simulink model "Bitwise_Testing"  (R2019a)
settings: Solver=FixedStepDiscrete  StartTime=0.0  StopTime=10.0  RelTol=1e-3
libraries: simulink x3
settings Model: Creator=Raouf  LastModifiedBy=Raouf
settings OptimizationCC: DefaultParameterBehavior=Inlined  EnhancedBackFolding=on  PassReuseOutputArgsAs=Individual arguments  OptimizeBlockOrder=speed  DifferentSizesBufferReuse=on  OptimizationCustomize=off
settings DebuggingCC: ParameterTunabilityLossMsg=error
settings SFSimCC: MATLABDynamicMemAlloc=off
settings RTWCC: SystemTargetFile=ert.tlc  GenCodeOnly=on  TemplateMakefile=ert_default_tmf  GenerateReport=on  IncludeHyperlinkInReport=on  LaunchReport=on  GenerateTraceInfo=on  GenerateTraceReport=on  GenerateTraceReportSl=on  GenerateTraceReportSf=on  GenerateTraceReportEml=on
settings CodeAppCC: ForceParamTrailComments=on  IgnoreCustomStorageClasses=off  OperatorAnnotations=on  SimulinkDataObjDesc=on  SFDataObjDesc=on  InsertBlockDesc=on
settings ERTTargetCC: TargetLangStandard=C99 (ISO)  GenerateSampleERTMain=on  InlinedParameterPlacement=NonHierarchical  ERTCustomFileTemplate=example_file_process.tlc

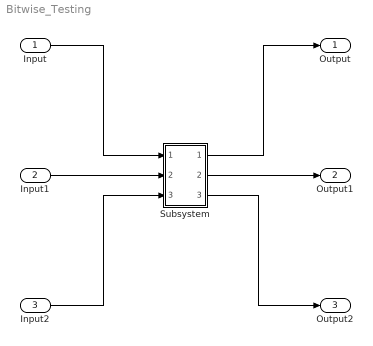
== system Bitwise_Testing ==
  Input : Inport  OutDataTypeStr=uint8
  Input1 : Inport  Port=2  OutDataTypeStr=uint8
  Input2 : Inport  Port=3  OutDataTypeStr=uint8
  Subsystem : Subsystem
  Output : Outport
  Output1 : Outport  Port=2
  Output2 : Outport  Port=3
  wires:
  Input/1 -> Subsystem/1(In1)
  Input1/1 -> Subsystem/2(In2)
  Input2/1 -> Subsystem/3(In3)
  Subsystem/1(Out1) -> Output/1
  Subsystem/2(Out2) -> Output1/1
  Subsystem/3(Out3) -> Output2/1

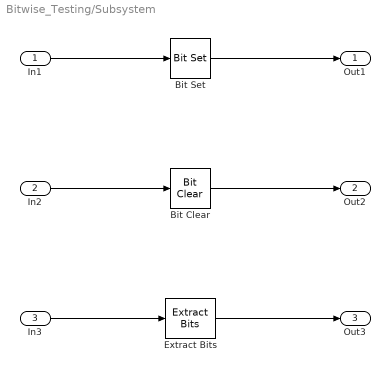
== system Bitwise_Testing/Subsystem ==
  In1 : Inport
  In2 : Inport  Port=2
  In3 : Inport  Port=3
  Bit Clear : simulink/Logic and Bit Operations/Bit Clear  iBit=0
      settings: SourceProductName=Simulink  SourceProductBaseCode=SL
  Bit Set : simulink/Logic and Bit Operations/Bit Set  iBit=0
      settings: SourceProductName=Simulink  SourceProductBaseCode=SL
  Extract Bits : simulink/Logic and Bit Operations/Extract Bits  bitsToExtract=Range of bits  numBits=[0 2]  bitIdxRange=[0 2]  outScalingMode=Treat bit field as an integer
      settings: SourceProductName=Simulink
  Out1 : Outport
  Out2 : Outport  Port=2
  Out3 : Outport  Port=3
  wires:
  Bit Set/1 -> Out1/1
  Extract Bits/1 -> Out3/1
  In2/1 -> Bit Clear/1
  In1/1 -> Bit Set/1
  In3/1 -> Extract Bits/1
  Bit Clear/1 -> Out2/1
